simulink model "sim_tcyb_2023_obs"  (R2020a)
settings: Solver=ode4  StartTime=0.0  StopTime=30.0  FixedStep=0.01  RelTol=1e-3
values from neighbouring files (symbols this model uses):
  b1 = 6.0    (= 6)    [init_tcyb_2023_obs.m]
  c1 = 6.0    (= 6)    [init_tcyb_2023_obs.m]
  delta1 = 0.1    [init_tcyb_2023_obs.m]
  delta2 = 0.1    [init_tcyb_2023_obs.m]
  k0 = 2    [init_tcyb_2023_obs.m]
  kai_1_t = 0.02    [init_tcyb_2023_obs.m]
  kai_3_t = 0.1    [init_tcyb_2023_obs.m]
  lambda_max_P = max(eig(Pij))    [init_tcyb_2023_obs.m]
  lambda_min_Q = min(eig(Qij))    [init_tcyb_2023_obs.m]
  Mii = diag([1;0;0;0;1])    [init_tcyb_2023_obs.m]
  pos0 = zeros(3, 1)    [init_tcyb_2023_obs.m]
  PZ0 = P0(3)    [init_tcyb_2023_obs.m]
  PZ1 = 10    [init_tcyb_2023_obs.m]
  R0 = 4    [init_tcyb_2023_obs.m]
  R1 = 8    [init_tcyb_2023_obs.m]
  Rx2 = 10    [init_tcyb_2023_obs.m]
  Ry2 = 6    [init_tcyb_2023_obs.m]
  Rz2 = 4    [init_tcyb_2023_obs.m]
  T0 = 0    [init_tcyb_2023_obs.m]
  T1 = tseq1    (= 10)    [init_tcyb_2023_obs.m]
  T12 = tseq1 + tseq12    (= 20)    [init_tcyb_2023_obs.m]
  T2 = tseq1 + tseq12 + tseq2    (= 30)    [init_tcyb_2023_obs.m]
  theta0 = ( 2 / 5 ) * pi    (= 1.25663706144)    [init_tcyb_2023_obs.m]
  ts1 = 10    [init_tcyb_2023_obs.m]
  ts2 = 20    [init_tcyb_2023_obs.m]
  vel0 = zeros(3, 1)    [init_tcyb_2023_obs.m]
  Wij = [0,0,1,0,0;              0,0,1,1,0;              1,0,0,0,1;              0,1,1,0,0;              0,0,1,0,0]    [init_tcyb_2023_obs.m]
  X1 = 8    [init_tcyb_2023_obs.m]
  X2 = 2    [init_tcyb_2023_obs.m]
  X3 = 3    [init_tcyb_2023_obs.m]
  Y1 = 10    [init_tcyb_2023_obs.m]
  Y2 = 2    [init_tcyb_2023_obs.m]
  Y3 = 4    [init_tcyb_2023_obs.m]
  Z1 = 4    [init_tcyb_2023_obs.m]
  Z2 = -6    [init_tcyb_2023_obs.m]
  Z3 = 2    [init_tcyb_2023_obs.m]
(part 1 of 2)
settings Model: Creator=zzy  LastModifiedBy=Hershey.A
settings DataIOCC: ReturnWorkspaceOutputs=off
settings DebuggingCC: ArithmeticOperatorsInVariantConditions=warning
settings SFSimCC: SimUseLocalCustomCode=off  CustomCodeUndefinedFunction=UseInterfaceOnly
settings RTWCC: RTWUseLocalCustomCode=off

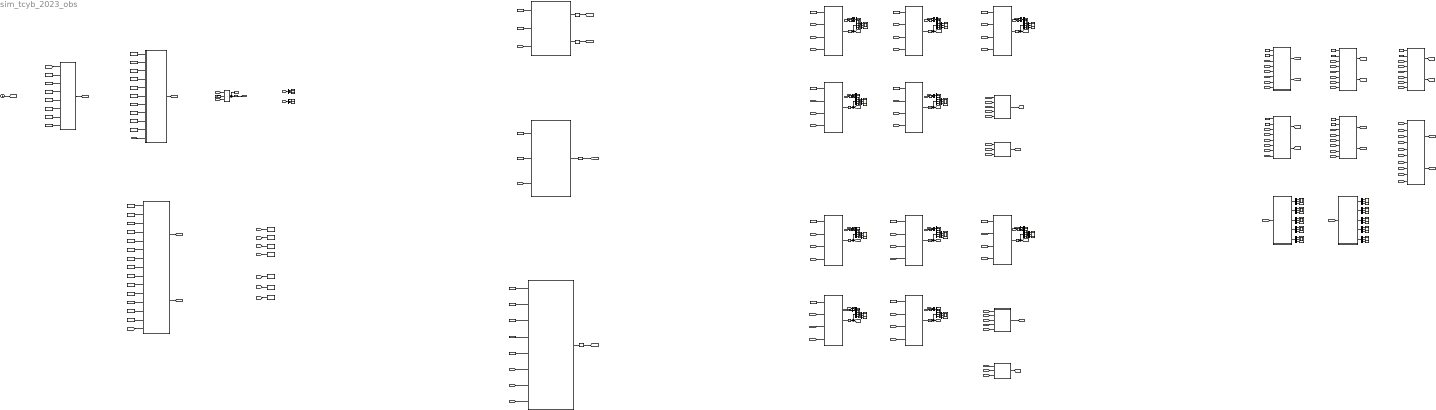
== system sim_tcyb_2023_obs ==
  Add{,1..9} (10 alike) : Sum
  Clock : Clock
  Constant : Constant  Value=T1
  Constant1 : Constant  Value=ts1
  Constant{10..14} (5 alike) : Constant  Value=c1
  Constant129 : Constant  Value=R0
  Constant130 : Constant  Value=R1
  Constant131 : Constant  Value=T0
  Constant132 : Constant  Value=Rz2
  Constant133 : Constant  Value=Ry2
  Constant134 : Constant  Value=Rx2
  Constant135 : Constant  Value=X1
  Constant136 : Constant  Value=X2
  Constant137 : Constant  Value=Y1
  Constant138 : Constant  Value=Y2
  Constant{15..19} (5 alike) : Constant  Value=b1
  Constant2 : Constant  Value=ts2
  Constant20 : Constant  Value=Z1
  Constant21 : Constant  Value=Z2
  Constant22 : Constant  Value=theta0
  Constant{223,227,232,236,240} (5 alike) : Constant  Value=Wij
  Constant{224,228,233,237,242} (5 alike) : Constant  Value=Mii
  Constant23 : Constant  Value=Z3
  Constant24 : Constant  Value=Y3
  Constant25 : Constant  Value=kai_1_t
  Constant26 : Constant  Value=X3
  Constant27 : Constant  Value=kai_3_t
  Constant28 : Constant  Value=T1
  Constant29 : Constant  Value=T12
  Constant3 : Constant  Value=k0
  Constant4 : Constant  Value=ts1
  Constant5 : Constant  Value=ts2
  Constant6 : Constant  Value=delta1
  Constant64 : Constant  Value=T2
  Constant65 : Constant  Value=R0
  Constant66 : Constant  Value=R1
  Constant67 : Constant  Value=Rx2
  Constant68 : Constant  Value=Ry2
  Constant69 : Constant  Value=Rz2
  Constant7 : Constant  Value=delta2
  Constant70 : Constant  Value=T2
  Constant71 : Constant  Value=T1
  Constant72 : Constant  Value=PZ0
  Constant73 : Constant  Value=PZ1
  Constant8 : Constant  Value=lambda_max_P
  Constant9 : Constant  Value=lambda_min_Q
  Demux{1,22,68..97} (32 alike) : Demux  Outputs=3
  Memory{,1..3} (4 alike) : Memory
  Mux{86..108,119,130..135} (30 alike) : Mux  Inputs=2
  Selector1 : Selector  NumberOfDimensions=2  InputPortWidth=3  IndexOptions=Index vector (dialog),Index vector (dialog)  Indices=[1 2 3],4  OutputSizes=1,1
  Selector10 : Selector  NumberOfDimensions=2  InputPortWidth=3  IndexOptions=Index vector (dialog),Index vector (dialog)  Indices=[1 2 3],5  OutputSizes=1,1
  Selector2 : Selector  NumberOfDimensions=2  InputPortWidth=3  IndexOptions=Index vector (dialog),Index vector (dialog)  Indices=[1 2 3],5  OutputSizes=1,1
  Selector3 : Selector  NumberOfDimensions=2  InputPortWidth=3  IndexOptions=Index vector (dialog),Index vector (dialog)  Indices=[1 2 3],3  OutputSizes=1,1
  Selector4 : Selector  NumberOfDimensions=2  InputPortWidth=3  IndexOptions=Index vector (dialog),Index vector (dialog)  Indices=[1 2 3],1  OutputSizes=1,1
  Selector5 : Selector  NumberOfDimensions=2  InputPortWidth=3  IndexOptions=Index vector (dialog),Index vector (dialog)  Indices=[1 2 3],2  OutputSizes=1,1
  Selector6 : Selector  NumberOfDimensions=2  InputPortWidth=3  IndexOptions=Index vector (dialog),Index vector (dialog)  Indices=[1 2 3],1  OutputSizes=1,1
  Selector7 : Selector  NumberOfDimensions=2  InputPortWidth=3  IndexOptions=Index vector (dialog),Index vector (dialog)  Indices=[1 2 3],2  OutputSizes=1,1
  Selector8 : Selector  NumberOfDimensions=2  InputPortWidth=3  IndexOptions=Index vector (dialog),Index vector (dialog)  Indices=[1 2 3],3  OutputSizes=1,1
  Selector9 : Selector  NumberOfDimensions=2  InputPortWidth=3  IndexOptions=Index vector (dialog),Index vector (dialog)  Indices=[1 2 3],4  OutputSizes=1,1
  Step : Step  Time=T1+0.01  SampleTime=0
  To Workspace : ToWorkspace  VariableName=eta_d_est_vec  SampleTime=-1
  To Workspace17 : ToWorkspace  VariableName=ksi_est_err  SampleTime=-1
  To Workspace18 : ToWorkspace  VariableName=ksi_d_est_vec  SampleTime=-1
  To Workspace22 : ToWorkspace  VariableName=eta_est_err  SampleTime=-1
  To Workspace3 : ToWorkspace  VariableName=u0  SampleTime=-1
  To Workspace4 : ToWorkspace  VariableName=eta0  SampleTime=-1
  To Workspace5 : ToWorkspace  VariableName=ksi0  SampleTime=-1
  cal lumped observation error agent 1 : MATLAB Function  TreatAsAtomicUnit=on
  cal lumped observation error agent 2 : MATLAB Function  TreatAsAtomicUnit=on
  cal lumped observation error agent 3 : MATLAB Function  TreatAsAtomicUnit=on
  cal lumped observation error agent 4 : MATLAB Function  TreatAsAtomicUnit=on
  cal lumped observation error agent 5 : MATLAB Function  TreatAsAtomicUnit=on
  cal position estimate error : MATLAB Function  TreatAsAtomicUnit=on
  cal velocity estimate error : MATLAB Function  TreatAsAtomicUnit=on
  combine follower desire velocity estimaters : MATLAB Function  TreatAsAtomicUnit=on
  combine leader position estimaters : MATLAB Function  TreatAsAtomicUnit=on
  "combine lumped follower observation error " : MATLAB Function  TreatAsAtomicUnit=on
  distributed follower desire position observer agent 1 : MATLAB Function  TreatAsAtomicUnit=on
  distributed follower desire position observer agent 2 : MATLAB Function  TreatAsAtomicUnit=on
  distributed follower desire position observer agent 3 : MATLAB Function  TreatAsAtomicUnit=on
  distributed follower desire position observer agent 4 : MATLAB Function  TreatAsAtomicUnit=on
  distributed follower desire position observer agent 5 : MATLAB Function  TreatAsAtomicUnit=on
  distributed follower desire velocity observer agent 1 : MATLAB Function  TreatAsAtomicUnit=on
  distributed follower desire velocity observer agent 2 : MATLAB Function  TreatAsAtomicUnit=on
  distributed follower desire velocity observer agent 3 : MATLAB Function  TreatAsAtomicUnit=on
  distributed follower desire velocity observer agent 4 : MATLAB Function  TreatAsAtomicUnit=on
  distributed follower desire velocity observer agent 5 : MATLAB Function  TreatAsAtomicUnit=on
  divide eta_est_err : MATLAB Function  TreatAsAtomicUnit=on
  divide ksi_est_err : MATLAB Function  TreatAsAtomicUnit=on
  eta_0 : Scope  NumInputPorts=3
  eta_d_est_{1..5} (5 alike) : Scope  NumInputPorts=3
  eta_est_err_{1..5} (5 alike) : Scope  NumInputPorts=3
  generate function eta_t : MATLAB Function  TreatAsAtomicUnit=on
  generate function h_t : MATLAB Function  TreatAsAtomicUnit=on
  generate function ksy_t d_ksy_t : MATLAB Function  TreatAsAtomicUnit=on
  ksi_0 : Scope  NumInputPorts=3
  ksi_d_est_{1..5} (5 alike) : Scope  NumInputPorts=3
  ksi_est_err_{1..5} (5 alike) : Scope  NumInputPorts=3
  leader control input : MATLAB Function  TreatAsAtomicUnit=on
  leader eta0 Integrator : Integrator  ExternalReset=rising  InitialConditionSource=external  InitialCondition=vel0
  leader ksi0 Integrator : Integrator  InitialCondition=pos0
  position observe Integrator {1..5} (5 alike) : Integrator  InitialCondition=zeros(3,1)
  process velocity : MATLAB Function  TreatAsAtomicUnit=on
  set desire formation configuration : MATLAB Function  TreatAsAtomicUnit=on
  velocity observe Integrator {1..5} (5 alike) : Integrator  InitialCondition=zeros(3,1)
  wires:
  [ksi0] -> cal lumped observation error agent 2/4(ksi0)
  Constant227/1 -> cal lumped observation error agent 2/1(wij)
  Add3/1 -> Demux76/1
  Add8/1 -> Demux97/1
  Mux134/1 -> ksi_d_est_3/2
  Mux135/1 -> ksi_d_est_3/3
  Demux93/2 -> Mux130/2
  position observe Integrator 2/1 -> [ksi_d_est_2], Demux92/1
  Demux95/3 -> Mux135/2
  [ksi0] -> cal lumped observation error agent 1/4(ksi0)
  Demux94/2 -> Mux134/1
  [ksi0] -> Add6/1
  velocity observe Integrator 5/1 -> [eta_d_est_5], Demux77/1
  Demux93/1 -> Mux119/2
  distributed follower desire position observer agent 2/1(d_ksi_d_est_2) -> position observe Integrator 2/1
  Demux93/3 -> Mux132/2
  Mux108/1 -> ksi_d_est_1/3
  Add6/1 -> Demux93/1
  Mux119/1 -> ksi_d_est_2/1
  Demux88/3 -> Mux108/2
  Demux88/1 -> Mux86/2
  Add5/1 -> Demux88/1
  [eta_est_err_tilt_3] -> "combine lumped follower observation error "/8(eta_est_err_tilt_3)
  Demux73/2 -> Mux100/1
  Add1/1 -> Demux72/1
  [ksi0] -> cal lumped observation error agent 3/4(ksi0)
  [eta_d_est_vec] -> cal lumped observation error agent 1/6(eta_d_est_vec)
  [ksi_est_err_tilt_4] -> "combine lumped follower observation error "/4(ksi_est_err_tilt_4)
  Mux103/1 -> eta_d_est_4/2
  velocity observe Integrator 4/1 -> [eta_d_est_4], Demux75/1
  Demux77/2 -> Mux106/1
  Demux77/1 -> Mux105/1
  Mux107/1 -> eta_d_est_5/3
  distributed follower desire velocity observer agent 5/1(d_eta_d_est_5) -> velocity observe Integrator 5/1
  Mux104/1 -> eta_d_est_4/3
  Demux74/3 -> Mux101/2
  distributed follower desire velocity observer agent 3/1(d_eta_d_est_3) -> velocity observe Integrator 3/1
  Demux74/2 -> Mux100/2
  Demux75/2 -> Mux103/1
  Demux76/3 -> Mux104/2
  Demux75/3 -> Mux104/1
  cal lumped observation error agent 4/2(eta_est_err_tilt_4) -> [eta_est_err_tilt_4]
  Mux95/1 -> eta_d_est_2/1
  velocity observe Integrator 3/1 -> [eta_d_est_3], Demux73/1
  velocity observe Integrator 2/1 -> [eta_d_est_2], Demux71/1
  Demux72/1 -> Mux95/2
  [eta0] -> Add2/1
  [eta_est_err_tilt_5] -> "combine lumped follower observation error "/10(eta_est_err_tilt_5)
  Add/1 -> Demux70/1
  cal lumped observation error agent 2/1(ksi_est_err_tilt_2) -> [ksi_est_err_tilt_2]
  distributed follower desire velocity observer agent 2/1(d_eta_d_est_2) -> velocity observe Integrator 2/1
  Mux98/1 -> eta_d_est_2/3
  [eta_d_est_5] -> combine follower desire velocity estimaters/5(eta_d_est_5)
  cal lumped observation error agent 3/1(ksi_est_err_tilt_3) -> [ksi_est_err_tilt_3]
  Demux72/2 -> Mux96/2
  [ksi_d_est_vec] -> cal lumped observation error agent 5/3(ksi_d_est_vec)
  [eta_d_est_2] -> combine follower desire velocity estimaters/2(eta_d_est_2)
  Constant228/1 -> cal lumped observation error agent 2/2(w0)
  [ksi_est_err_tilt_2] -> "combine lumped follower observation error "/2(ksi_est_err_tilt_2)
  [ksi_est_err_tilt_5] -> "combine lumped follower observation error "/5(ksi_est_err_tilt_5)
  Demux76/1 -> Mux102/2
  cal lumped observation error agent 5/1(ksi_est_err_tilt_5) -> [ksi_est_err_tilt_5]
  [eta_est_err_tilt_2] -> "combine lumped follower observation error "/7(eta_est_err_tilt_2)
  [ksi_d_est_vec] -> cal lumped observation error agent 3/3(ksi_d_est_vec)
  Constant242/1 -> cal lumped observation error agent 5/2(w0)
  [ksi_d_est_vec] -> cal lumped observation error agent 4/3(ksi_d_est_vec)
  Mux105/1 -> eta_d_est_5/1
  [eta_est_err_tilt_4] -> "combine lumped follower observation error "/9(eta_est_err_tilt_4)
  Add7/1 -> Demux95/1
  Constant236/1 -> cal lumped observation error agent 4/1(wij)
  [eta0] -> cal lumped observation error agent 1/7(eta0)
  [eta0] -> cal lumped observation error agent 2/7(eta0)
  cal lumped observation error agent 1/2(eta_est_err_tilt_1) -> [eta_est_err_tilt_1]
  Demux77/3 -> Mux107/1
  cal lumped observation error agent 1/1(ksi_est_err_tilt_1) -> [ksi_est_err_tilt_1]
  [eta_d_est_vec] -> cal lumped observation error agent 2/6(eta_d_est_vec)
  cal lumped observation error agent 4/1(ksi_est_err_tilt_4) -> [ksi_est_err_tilt_4]
  Mux93/1 -> eta_d_est_1/2
  Demux69/2 -> Mux93/1
  Mux100/1 -> eta_d_est_3/2
  Mux94/1 -> eta_d_est_1/3
  Demux73/1 -> Mux99/1
  [ksi_d_est_3] -> combine leader position estimaters/3(ksi_d_est_3)
  Demux70/2 -> Mux93/2
  [eta0] -> Add/1
  [ksi0] -> cal position estimate error/2(ksi0)
  Demux69/3 -> Mux94/1
  distributed follower desire position observer agent 3/1(d_ksi_d_est_3) -> position observe Integrator 3/1
  [eta_d_est_4] -> combine follower desire velocity estimaters/4(eta_d_est_4)
  [eta_d_est_1] -> combine follower desire velocity estimaters/1(eta_d_est_1)
  Constant233/1 -> cal lumped observation error agent 3/2(w0)
  Demux78/1 -> Mux86/1
  Demux86/3 -> eta_est_err_1/3
  Demux89/2 -> eta_est_err_3/2
  Demux87/1 -> eta_est_err_2/1
  divide eta_est_err/2(eta_est_err_2) -> Demux87/1
  Demux85/2 -> ksi_est_err_5/2
  Demux90/1 -> eta_est_err_4/1
  Demux90/2 -> eta_est_err_4/2
  Mux86/1 -> ksi_d_est_1/1
  Mux130/1 -> ksi_d_est_2/2
  Demux87/2 -> eta_est_err_2/2
  Mux131/1 -> ksi_d_est_5/3
  distributed follower desire position observer agent 1/1(d_ksi_d_est_1) -> position observe Integrator 1/1
  Demux84/1 -> ksi_est_err_4/1
  divide eta_est_err/4(eta_est_err_4) -> Demux90/1
  position observe Integrator 5/1 -> [ksi_d_est_5], Demux68/1
  Demux85/3 -> ksi_est_err_5/3
  Constant224/1 -> cal lumped observation error agent 1/2(w0)
  Demux85/1 -> ksi_est_err_5/1
  Mux97/1 -> ksi_d_est_1/2
  Demux84/2 -> ksi_est_err_4/2
  Demux94/3 -> Mux135/1
  divide ksi_est_err/4(ksi_est_err_4) -> Demux84/1
  Mux89/1 -> ksi_d_est_4/3
  Demux82/3 -> ksi_est_err_2/3
  Demux92/2 -> Mux130/1
  Constant240/1 -> cal lumped observation error agent 5/1(wij)
  [eta0] -> Add3/1
  Demux83/3 -> ksi_est_err_3/3
  Demux86/2 -> eta_est_err_1/2
  Demux88/2 -> Mux97/2
  Demux81/1 -> ksi_est_err_1/1
  Demux82/2 -> ksi_est_err_2/2
  [ksi_d_est_5] -> combine leader position estimaters/5(ksi_d_est_5)
  divide ksi_est_err/2(ksi_est_err_2) -> Demux82/1
  Demux91/1 -> eta_est_err_5/1
  position observe Integrator 3/1 -> [ksi_d_est_3], Demux94/1
  divide ksi_est_err/1(ksi_est_err_1) -> Demux81/1
  Demux82/1 -> ksi_est_err_2/1
  Demux68/3 -> Mux131/1
  distributed follower desire position observer agent 5/1(d_ksi_d_est_5) -> position observe Integrator 5/1
  Demux78/2 -> Mux97/1
  [eta0] -> cal lumped observation error agent 5/7(eta0)
  Demux78/3 -> Mux108/1
  [eta_d_est_3] -> combine follower desire velocity estimaters/3(eta_d_est_3)
  [eta0] -> cal velocity estimate error/2(eta0)
  Mux91/1 -> ksi_d_est_5/2
  Demux71/2 -> Mux96/1
  [eta_d_est_vec] -> cal lumped observation error agent 5/6(eta_d_est_vec)
  [ksi0] -> Add7/1
  [ksi0] -> Add9/1
  [ksi_est_err_tilt_1] -> "combine lumped follower observation error "/1(ksi_est_err_tilt_1)
  distributed follower desire velocity observer agent 4/1(d_eta_d_est_4) -> velocity observe Integrator 4/1
  Mux90/1 -> ksi_d_est_5/1
  Constant223/1 -> cal lumped observation error agent 1/1(wij)
  [eta0] -> cal lumped observation error agent 3/7(eta0)
  Demux80/1 -> Mux90/2
  Mux88/1 -> ksi_d_est_4/2
  Add4/1 -> Demux79/1
  Constant232/1 -> cal lumped observation error agent 3/1(wij)
  Mux87/1 -> ksi_d_est_4/1
  position observe Integrator 1/1 -> [ksi_d_est_1], Demux78/1
  Demux80/3 -> Mux131/2
  [ksi0] -> cal lumped observation error agent 5/4(ksi0)
  [ksi_d_est_vec] -> cal position estimate error/1(ksi_d_est_vec)
  Demux73/3 -> Mux101/1
  Demux69/1 -> Mux92/1
  Demux96/2 -> Mux88/1
  position observe Integrator 4/1 -> [ksi_d_est_4], Demux96/1
  Demux72/3 -> Mux98/2
  Demux74/1 -> Mux99/2
  Constant237/1 -> cal lumped observation error agent 4/2(w0)
  Mux132/1 -> ksi_d_est_2/3
  Demux70/3 -> Mux94/2
  Demux71/1 -> Mux95/1
  Mux133/1 -> ksi_d_est_3/1
  [ksi0] -> Add8/1
  cal lumped observation error agent 3/2(eta_est_err_tilt_3) -> [eta_est_err_tilt_3]
  distributed follower desire position observer agent 4/1(d_ksi_d_est_4) -> position observe Integrator 4/1
  [eta_d_est_vec] -> cal velocity estimate error/1(eta_d_est_vec)
  Add2/1 -> Demux74/1
  Demux95/2 -> Mux134/2
  Demux97/1 -> Mux87/2
  [eta0] -> Add1/1
  [eta0] -> Add4/1
  [ksi0] -> cal lumped observation error agent 4/4(ksi0)
  distributed follower desire velocity observer agent 1/1(d_eta_d_est_1) -> velocity observe Integrator 1/1
  Demux96/1 -> Mux87/1
  [ksi_d_est_2] -> combine leader position estimaters/2(ksi_d_est_2)
  [ksi_d_est_vec] -> cal lumped observation error agent 1/3(ksi_d_est_vec)
  Demux97/2 -> Mux88/2
  Demux83/2 -> ksi_est_err_3/2
  [ksi_est_err_tilt_3] -> "combine lumped follower observation error "/3(ksi_est_err_tilt_3)
  Demux71/3 -> Mux98/1
  Demux86/1 -> eta_est_err_1/1
  Mux101/1 -> eta_d_est_3/3
  cal lumped observation error agent 2/2(eta_est_err_tilt_2) -> [eta_est_err_tilt_2]
  Demux87/3 -> eta_est_err_2/3
  Mux96/1 -> eta_d_est_2/2
  Demux79/3 -> Mux107/2
  cal lumped observation error agent 5/2(eta_est_err_tilt_5) -> [eta_est_err_tilt_5]
  [eta_est_err] -> divide eta_est_err/1(eta_est_err)
  velocity observe Integrator 1/1 -> [eta_d_est_1], Demux69/1
  [ksi_d_est_4] -> combine leader position estimaters/4(ksi_d_est_4)
  Demux76/2 -> Mux103/2
  Demux79/2 -> Mux106/2
  [eta0] -> cal lumped observation error agent 4/7(eta0)
  divide ksi_est_err/3(ksi_est_err_3) -> Demux83/1
  Demux95/1 -> Mux133/2
  divide eta_est_err/5(eta_est_err_5) -> Demux91/1
  Demux96/3 -> Mux89/1
  Demux92/1 -> Mux119/1
  Mux99/1 -> eta_d_est_3/1
  Demux89/1 -> eta_est_err_3/1
  Demux83/1 -> ksi_est_err_3/1
  Demux81/3 -> ksi_est_err_1/3
  Add9/1 -> Demux80/1
  Mux102/1 -> eta_d_est_4/1
  Demux68/1 -> Mux90/1
  Demux80/2 -> Mux91/2
  Demux92/3 -> Mux132/1
  [eta_est_err_tilt_1] -> "combine lumped follower observation error "/6(eta_est_err_tilt_1)
  [ksi_est_err] -> divide ksi_est_err/1(ksi_est_err)
  Demux68/2 -> Mux91/1
  Demux91/3 -> eta_est_err_5/3
  [ksi0] -> Add5/1
  [ksi_d_est_1] -> combine leader position estimaters/1(ksi_d_est_1)
  [ksi_d_est_vec] -> cal lumped observation error agent 2/3(ksi_d_est_vec)
  Demux94/1 -> Mux133/1
  divide eta_est_err/3(eta_est_err_3) -> Demux89/1
  Demux89/3 -> eta_est_err_3/3
  divide ksi_est_err/5(ksi_est_err_5) -> Demux85/1
  Demux79/1 -> Mux105/2
  [eta_d_est_vec] -> cal lumped observation error agent 3/6(eta_d_est_vec)
  Demux81/2 -> ksi_est_err_1/2
  Demux84/3 -> ksi_est_err_4/3
  Demux70/1 -> Mux92/2
  Demux91/2 -> eta_est_err_5/2
  Demux90/3 -> eta_est_err_4/3
  [eta_d_est_vec] -> cal lumped observation error agent 4/6(eta_d_est_vec)
  Demux75/1 -> Mux102/1
  divide eta_est_err/1(eta_est_err_1) -> Demux86/1
  Mux106/1 -> eta_d_est_5/2
  Demux97/3 -> Mux89/2
  Mux92/1 -> eta_d_est_1/1
  cal position estimate error/1(ksi_est_err) -> [ksi_est_err]
  cal velocity estimate error/1(eta_est_err) -> [eta_est_err]
  combine leader position estimaters/1(ksi_d_est_vec) -> [ksi_d_est_vec]
  combine follower desire velocity estimaters/1(eta_d_est_vec) -> [eta_d_est_vec]
  "combine lumped follower observation error "/1(ksi_est_err_tilt_vec) -> [ksi_est_err_tilt_vec]
  "combine lumped follower observation error "/2(eta_est_err_tilt_vec) -> [eta_est_err_tilt_vec]
  [tsim] -> generate function ksy_t d_ksy_t/3(tsim)
  Constant1/1 -> generate function ksy_t d_ksy_t/1(ts1)
  Constant2/1 -> generate function ksy_t d_ksy_t/2(ts2)
  generate function ksy_t d_ksy_t/1(ksy_t) -> Memory/1
  Memory/1 -> [ksy_t]
  Memory1/1 -> [d_ksy_t]
  generate function ksy_t d_ksy_t/2(d_ksy_t) -> Memory1/1
  Constant3/1 -> generate function h_t/1(k0)
  Constant4/1 -> generate function h_t/2(ts1)
  Constant5/1 -> generate function h_t/3(ts2)
  [tsim] -> generate function h_t/6(tsim)
  Constant6/1 -> generate function h_t/4(delta1)
  Constant7/1 -> generate function h_t/5(delta2)
  [ksy_t] -> generate function h_t/7(ksy_t)
  [d_ksy_t] -> generate function h_t/8(d_ksy_t)
  Memory2/1 -> [h_t]
  generate function h_t/1(h_t) -> Memory2/1
  Constant8/1 -> generate function eta_t/1(lambda_max_P)
  Constant9/1 -> generate function eta_t/2(lambda_min_Q)
  [h_t] -> generate function eta_t/3(h_t)
  Memory3/1 -> [eta_t]
  generate function eta_t/1(eta_t) -> Memory3/1
  Constant10/1 -> distributed follower desire velocity observer agent 1/1(c1)
  [eta_t] -> distributed follower desire velocity observer agent 1/2(eta_t)
  [eta_est_err_tilt_vec] -> distributed follower desire velocity observer agent 1/4(eta_est_err_tilt_vec)
  Constant11/1 -> distributed follower desire velocity observer agent 2/1(c1)
  [eta_t] -> distributed follower desire velocity observer agent 2/2(eta_t)
  [eta_est_err_tilt_vec] -> distributed follower desire velocity observer agent 2/4(eta_est_err_tilt_vec)
  [eta_est_err_tilt_vec] -> distributed follower desire velocity observer agent 3/4(eta_est_err_tilt_vec)
  [eta_t] -> distributed follower desire velocity observer agent 3/2(eta_t)
  Constant12/1 -> distributed follower desire velocity observer agent 3/1(c1)
  Constant13/1 -> distributed follower desire velocity observer agent 4/1(c1)
  [eta_t] -> distributed follower desire velocity observer agent 4/2(eta_t)
  [eta_est_err_tilt_vec] -> distributed follower desire velocity observer agent 4/4(eta_est_err_tilt_vec)
  Constant14/1 -> distributed follower desire velocity observer agent 5/1(c1)
  [eta_t] -> distributed follower desire velocity observer agent 5/2(eta_t)
  [eta_est_err_tilt_vec] -> distributed follower desire velocity observer agent 5/4(eta_est_err_tilt_vec)
  Constant15/1 -> distributed follower desire position observer agent 1/1(b1)
  [ksi_est_err_tilt_vec] -> distributed follower desire position observer agent 1/3(ksi_est_err_tilt_vec)
  [eta_t] -> distributed follower desire position observer agent 1/2(eta_t)
  [eta_d_est_vec] -> distributed follower desire position observer agent 1/4(eta_d_est_vec)
  Constant16/1 -> distributed follower desire position observer agent 2/1(b1)
  [eta_t] -> distributed follower desire position observer agent 2/2(eta_t)
  [ksi_est_err_tilt_vec] -> distributed follower desire position observer agent 2/3(ksi_est_err_tilt_vec)
  [eta_d_est_vec] -> distributed follower desire position observer agent 2/4(eta_d_est_vec)
  Constant17/1 -> distributed follower desire position observer agent 3/1(b1)
  [eta_t] -> distributed follower desire position observer agent 3/2(eta_t)
  [ksi_est_err_tilt_vec] -> distributed follower desire position observer agent 3/3(ksi_est_err_tilt_vec)
  [eta_d_est_vec] -> distributed follower desire position observer agent 3/4(eta_d_est_vec)
  Constant18/1 -> distributed follower desire position observer agent 4/1(b1)
  [eta_t] -> distributed follower desire position observer agent 4/2(eta_t)
  [ksi_est_err_tilt_vec] -> distributed follower desire position observer agent 4/3(ksi_est_err_tilt_vec)
  [eta_d_est_vec] -> distributed follower desire position observer agent 4/4(eta_d_est_vec)
  Constant19/1 -> distributed follower desire position observer agent 5/1(b1)
  [eta_t] -> distributed follower desire position observer agent 5/2(eta_t)
  [ksi_est_err_tilt_vec] -> distributed follower desire position observer agent 5/3(ksi_est_err_tilt_vec)
  [eta_d_est_vec] -> distributed follower desire position observer agent 5/4(eta_d_est_vec)
  Selector2/1 -> Add4/2
  [delta_eta_vec] -> Selector2/1
  [delta_eta_vec] -> Selector1/1
  Selector1/1 -> Add3/2
  [delta_eta_vec] -> Selector3/1
  Selector3/1 -> Add2/2
  [delta_eta_vec] -> Selector4/1
  Selector4/1 -> Add/2
  [delta_eta_vec] -> Selector5/1
  Selector5/1 -> Add1/2
  Constant28/1 -> set desire formation configuration/13(T1)
  Constant72/1 -> process velocity/4(PZ0)
  leader ksi0 Integrator/1 -> [ksi0]
  Constant70/1 -> process velocity/3(T2)
  [tsim] -> set desire formation configuration/15(t)
  Constant20/1 -> set desire formation configuration/7(Z1)
  [tsim] -> leader control input/1(t)
  Step/1 -> leader eta0 Integrator/2
  Demux1/2 -> ksi_0/2
  Constant129/1 -> process velocity/6(R0)
  Constant/1 -> leader control input/2(T1)
  Constant22/1 -> set desire formation configuration/10(theta0)
  set desire formation configuration/2(delta_eta_vec) -> [delta_eta_vec]
  Constant71/1 -> process velocity/2(T1)
  Constant138/1 -> set desire formation configuration/5(Y2)
  Constant21/1 -> set desire formation configuration/8(Z2)
  set desire formation configuration/1(delta_ksi_vec) -> [delta_ksi_vec]
  Constant24/1 -> set desire formation configuration/6(Y3)
  Constant132/1 -> process velocity/10(Rz2)
  Demux22/1 -> eta_0/1
  [V_init_out] -> leader eta0 Integrator/3
  Constant68/1 -> leader control input/7(Ry2)
  Demux1/3 -> ksi_0/3
  Constant25/1 -> set desire formation configuration/11(kai_1_t)
  Demux22/2 -> eta_0/2
  Constant29/1 -> set desire formation configuration/14(T12)
  [tsim] -> process velocity/11(t)
  Constant135/1 -> set desire formation configuration/1(X1)
  Constant23/1 -> set desire formation configuration/9(Z3)
  [eta0] -> Demux22/1
  Constant133/1 -> process velocity/9(Ry2)
  Constant73/1 -> process velocity/5(PZ1)
  Demux1/1 -> ksi_0/1
  process velocity/1(V_init_out) -> [V_init_out]
  Demux22/3 -> eta_0/3
  Constant65/1 -> leader control input/4(R0)
  leader eta0 Integrator/1 -> [eta0], leader ksi0 Integrator/1
  Constant67/1 -> leader control input/6(Rx2)
  [ksi0] -> Demux1/1
  Clock/1 -> [tsim]
  Constant131/1 -> process velocity/1(T0)
  Constant137/1 -> set desire formation configuration/4(Y1)
  leader control input/1(u0) -> [u0]
  Constant64/1 -> leader control input/3(T2)
  Constant130/1 -> process velocity/7(R1)
  [u0] -> leader eta0 Integrator/1
  Constant134/1 -> process velocity/8(Rx2)
  Constant26/1 -> set desire formation configuration/3(X3)
  Constant66/1 -> leader control input/5(R1)
  Constant27/1 -> set desire formation configuration/12(kai_3_t)
  Constant69/1 -> leader control input/8(Rz2)
  Constant136/1 -> set desire formation configuration/2(X2)
  [ksi_est_err] -> To Workspace17/1
  [u0] -> To Workspace3/1
  [eta_est_err] -> To Workspace22/1
  [ksi_d_est_vec] -> To Workspace18/1
  [ksi0] -> To Workspace5/1
  [eta_d_est_vec] -> To Workspace/1
  [eta0] -> To Workspace4/1
  [delta_ksi_vec] -> cal lumped observation error agent 2/5(delta_ksi_vec)
  [delta_ksi_vec] -> Selector6/1
  Selector6/1 -> Add5/2
  [delta_ksi_vec] -> Selector7/1
  Selector7/1 -> Add6/2
  [delta_ksi_vec] -> Selector8/1
  Selector8/1 -> Add7/2
  [delta_ksi_vec] -> Selector9/1
  Selector9/1 -> Add8/2
  [delta_ksi_vec] -> Selector10/1
  Selector10/1 -> Add9/2
  [delta_ksi_vec] -> cal lumped observation error agent 1/5(delta_ksi_vec)
  [delta_eta_vec] -> cal lumped observation error agent 1/8(delta_eta_vec)
  [delta_ksi_vec] -> cal lumped observation error agent 3/5(delta_ksi_vec)
  [delta_eta_vec] -> cal lumped observation error agent 3/8(delta_eta_vec)
  [delta_ksi_vec] -> cal lumped observation error agent 5/5(delta_ksi_vec)
  [delta_eta_vec] -> cal lumped observation error agent 5/8(delta_eta_vec)
  [delta_eta_vec] -> cal lumped observation error agent 2/8(delta_eta_vec)
  [delta_ksi_vec] -> cal lumped observation error agent 4/5(delta_ksi_vec)
  [delta_eta_vec] -> cal lumped observation error agent 4/8(delta_eta_vec)
  [u0] -> distributed follower desire velocity observer agent 1/3(u0)
  [u0] -> distributed follower desire velocity observer agent 2/3(u0)
  [u0] -> distributed follower desire velocity observer agent 3/3(u0)
  [u0] -> distributed follower desire velocity observer agent 4/3(u0)
  [u0] -> distributed follower desire velocity observer agent 5/3(u0)
  [delta_ksi_vec] -> cal position estimate error/3(delta_ksi_vec)
  [delta_eta_vec] -> cal velocity estimate error/3(delta_eta_vec)

== matlab function sim_tcyb_2023_obs/set desire formation configuration ==
  data: X1 input; X2 input; X3 input; Y1 input; Y2 input; Y3 input; Z1 input; Z2 input; Z3 input; theta0 input; kai_1_t input; kai_3_t input; T1 input; T12 input; t input; delta_ksi_vec output; delta_eta_vec output
function [delta_ksi_vec, delta_eta_vec] = fcn(X1, X2, X3, Y1, Y2, Y3, Z1, Z2, Z3, theta0, ...
                                                                                    kai_1_t, kai_3_t, T1, T12, t)
%%%% 计算跟随者期望速度分布式观测器误差
delta_ksi_vec = zeros(3, 5);
delta_eta_vec = zeros(3, 5);
if t <= ( T1 + 1e-04 )
    exp_tmp = exp( -kai_1_t * t );
    delta_ksi_vec(:, 1) = [ X1 * cos( theta0 ) - X2 * exp_tmp; ...
                                            Y1 * sin( theta0 ) - Y2 * exp_tmp; ...
                                            Z1 - Z2 * exp_tmp ];
    delta_ksi_vec(:, 2) = [ - X1 * cos( theta0 ) + X2 * exp_tmp; ...
                                            Y1 * sin( theta0 ) - Y2 * exp_tmp; ...
                                            Z1 + Z2 * exp_tmp ];
    delta_ksi_vec(:, 3) = [ X1 - X2 * exp_tmp; ...
                                            Y2 * exp_tmp; ...
                                            ( 3 / 8 ) * Z1 + Z2 * exp_tmp ];
    delta_ksi_vec(:, 4) = [ - X1 * cos( theta0 ) + X2 * exp_tmp; ...
                                            - Y1 * sin( theta0 ) + Y2 * exp_tmp; ...
                                            Z1 + Z2 * exp_tmp ];
    delta_ksi_vec(:, 5) = [ X1 * cos( theta0 ) - X2 * exp_tmp; ...
                                            - Y1 * sin( theta0 ) + Y2 * exp_tmp; ...
                                            Z1 - Z2 * exp_tmp ];
    delta_eta_vec(:, 1) = [ kai_1_t * X2 * exp_tmp; kai_1_t * Y2 * exp_tmp; kai_1_t * Z2 * exp_tmp ];
    delta_eta_vec(:, 2) = [ - kai_1_t * X2 * exp_tmp; kai_1_t * Y2 * exp_tmp; - kai_1_t * Z2 * exp_tmp ];
    delta_eta_vec(:, 3) = [ kai_1_t * X2 * exp_tmp; - kai_1_t * Y2 * exp_tmp; - kai_1_t * Z2 * exp_tmp ];
    delta_eta_vec(:, 4) = [ - kai_1_t * X2 * exp_tmp; - kai_1_t * Y2 * exp_tmp; - kai_1_t * Z2 * exp_tmp ];
    delta_eta_vec(:, 5) = [ kai_1_t * X2 * exp_tmp; - kai_1_t * Y2 * exp_tmp; kai_1_t * Z2 * exp_tmp ];
elseif t <= ( T12 + 1e-04 )
    delta_ksi_vec(:, 1) = [ X1 * cos( theta0 ) - X2; Y1 * sin( theta0 ) - Y2; Z1 - Z2 ];
    delta_ksi_vec(:, 2) = [ - X1 * cos( theta0 ) + X2; Y1 * sin( theta0 ) - Y2; Z1 + Z2 ];
    delta_ksi_vec(:, 3) = [ X1 - X2; 0; ( 3 / 8 ) * Z1 + Z2 ];
    delta_ksi_vec(:, 4) = [ - X1 * cos( theta0 ) + X2; - Y1 * sin( theta0 ) + Y2; Z1 + Z2 ];
    delta_ksi_vec(:, 5) = [ X1 * cos( theta0 ) - X2; - Y1 * sin( theta0 ) + Y2; Z1 - Z2 ];
else
    exp_tmp = 1 / ( 1 + exp( - kai_3_t * ( t - T12 - 5 ) ) );
    tmp_2 = exp( - kai_3_t * ( t - T12 - 5 ) ) / ( ( 1 + exp( - kai_3_t * ( t - T12 - 5 ) ) ) ^ 2 );
    delta_ksi_vec(:, 1) = [ X1 * cos( theta0 ) - X2 + X3 * exp_tmp; ...
                                            Y1 * sin( theta0 ) - Y2 + Y3 * exp_tmp; ...
                                            Z1 - Z2 + Z3 * exp_tmp ];
    delta_ksi_vec(:, 2) = [ - X1 * cos( theta0 ) + X2 - X3 * exp_tmp; ...
                                            Y1 * sin( theta0 ) - Y2 + Y3 * exp_tmp; ...
                                            Z1 + Z2 - Z3 * exp_tmp ];
    delta_ksi_vec(:, 3) = [ X1 - X2 + X3 * exp_tmp; ...
                                            - Y3 * exp_tmp; ...
                                            ( 3 / 8 ) * Z1 + Z2 - Z3 * exp_tmp ];
    delta_ksi_vec(:, 4) = [ - X1 * cos( theta0 ) + X2 - X3 * exp_tmp; ...
                                            - Y1 * sin( theta0 ) + Y2 - Y3 * exp_tmp; ...
                                            Z1 + Z2 - Z3 * exp_tmp ];
    delta_ksi_vec(:, 5) = [ X1 * cos( theta0 ) - X2 + X3 * exp_tmp; ...
                                            - Y1 * sin( theta0 ) + Y2 - Y3 * exp_tmp; ...
                                            Z1 - Z2 + Z3 * exp_tmp ];
    delta_eta_vec(:, 1) = [ kai_3_t * X3 * tmp_2; kai_3_t * Y3 * tmp_2; kai_3_t * Z3 * tmp_2 ];
    delta_eta_vec(:, 2) = [ - kai_3_t * X3 * tmp_2; kai_3_t * Y3 * tmp_2; kai_3_t * Z3 * tmp_2 ];
    delta_eta_vec(:, 3) = [ kai_3_t * X3 * tmp_2; - kai_3_t * Y3 * tmp_2; - kai_3_t * Z3 * tmp_2 ];
    delta_eta_vec(:, 4) = [ - kai_3_t * X3 * tmp_2; - kai_3_t * Y3 * tmp_2; - kai_3_t * Z3 * tmp_2 ];
    delta_eta_vec(:, 5) = [ kai_3_t * X3 * tmp_2; kai_3_t * Y3 * tmp_2; - kai_3_t * Z3 * tmp_2 ];
end

== matlab function sim_tcyb_2023_obs/distributed follower desire velocity observer agent 2 ==
  data: c1 input; d_eta_d_est_2 output; eta_t input; u0 input; eta_est_err_tilt_vec input
function d_eta_d_est_2 = fcn(c1, eta_t, u0, eta_est_err_tilt_vec)
%%%% 跟随者期望速度分布式观测器
iiuav = 2;
d_eta_d_est_2 = u0(:) - 2 * ( eta_t + 2 ) * eta_est_err_tilt_vec(:,iiuav) ...
                                - c1 * ( eta_t + 2 ) * sign( eta_est_err_tilt_vec(:,iiuav) );

== matlab function sim_tcyb_2023_obs/distributed follower desire velocity observer agent 3 ==
  data: c1 input; d_eta_d_est_3 output; eta_t input; u0 input; eta_est_err_tilt_vec input
function d_eta_d_est_3 = fcn(c1, eta_t, u0, eta_est_err_tilt_vec)
%%%% 跟随者期望速度分布式观测器
iiuav = 3;
d_eta_d_est_3 = u0(:) - 2 * ( eta_t + 2 ) * eta_est_err_tilt_vec(:,iiuav) ...
                                - c1 * ( eta_t + 2 ) * sign( eta_est_err_tilt_vec(:,iiuav) );

== matlab function sim_tcyb_2023_obs/distributed follower desire velocity observer agent 4 ==
  data: c1 input; d_eta_d_est_4 output; eta_t input; u0 input; eta_est_err_tilt_vec input
function d_eta_d_est_4 = fcn(c1, eta_t, u0, eta_est_err_tilt_vec)
%%%% 跟随者期望速度分布式观测器
iiuav = 4;
d_eta_d_est_4 = u0(:) - 2 * ( eta_t + 2 ) * eta_est_err_tilt_vec(:,iiuav) ...
                                - c1 * ( eta_t + 2 ) * sign( eta_est_err_tilt_vec(:,iiuav) );

== matlab function sim_tcyb_2023_obs/distributed follower desire velocity observer agent 5 ==
  data: c1 input; d_eta_d_est_5 output; eta_t input; u0 input; eta_est_err_tilt_vec input
function d_eta_d_est_5 = fcn(c1, eta_t, u0, eta_est_err_tilt_vec)
%%%% 跟随者期望速度分布式观测器
iiuav = 5;
d_eta_d_est_5 = u0(:) - 2 * ( eta_t + 2 ) * eta_est_err_tilt_vec(:,iiuav) ...
                                - c1 * ( eta_t + 2 ) * sign( eta_est_err_tilt_vec(:,iiuav) );

== matlab function sim_tcyb_2023_obs/distributed follower desire position observer agent 1 ==
  data: b1 input; d_ksi_d_est_1 output; eta_t input; ksi_est_err_tilt_vec input; eta_d_est_vec input
function d_ksi_d_est_1 = fcn(b1, eta_t, ksi_est_err_tilt_vec, eta_d_est_vec)
%%%% 跟随者期望速度分布式观测器
iiuav = 1;
d_ksi_d_est_1 = eta_d_est_vec(:,iiuav) - 2 * ( eta_t + 2 ) * ksi_est_err_tilt_vec(:,iiuav) ...
                                - b1 * ( eta_t + 2 ) * sign( ksi_est_err_tilt_vec(:,iiuav) );

== matlab function sim_tcyb_2023_obs/distributed follower desire position observer agent 2 ==
  data: b1 input; d_ksi_d_est_2 output; eta_t input; ksi_est_err_tilt_vec input; eta_d_est_vec input
function d_ksi_d_est_2 = fcn(b1, eta_t, ksi_est_err_tilt_vec, eta_d_est_vec)
%%%% 跟随者期望速度分布式观测器
iiuav = 2;
d_ksi_d_est_2 = eta_d_est_vec(:,iiuav) - 2 * ( eta_t + 2 ) * ksi_est_err_tilt_vec(:,iiuav) ...
                                - b1 * ( eta_t + 2 ) * sign( ksi_est_err_tilt_vec(:,iiuav) );

== matlab function sim_tcyb_2023_obs/distributed follower desire position observer agent 3 ==
  data: b1 input; d_ksi_d_est_3 output; eta_t input; ksi_est_err_tilt_vec input; eta_d_est_vec input
function d_ksi_d_est_3 = fcn(b1, eta_t, ksi_est_err_tilt_vec, eta_d_est_vec)
%%%% 跟随者期望速度分布式观测器
iiuav = 3;
d_ksi_d_est_3 = eta_d_est_vec(:,iiuav) - 2 * ( eta_t + 2 ) * ksi_est_err_tilt_vec(:,iiuav) ...
                                - b1 * ( eta_t + 2 ) * sign( ksi_est_err_tilt_vec(:,iiuav) );

== matlab function sim_tcyb_2023_obs/distributed follower desire position observer agent 4 ==
  data: b1 input; d_ksi_d_est_4 output; eta_t input; ksi_est_err_tilt_vec input; eta_d_est_vec input
function d_ksi_d_est_4 = fcn(b1, eta_t, ksi_est_err_tilt_vec, eta_d_est_vec)
%%%% 跟随者期望速度分布式观测器
iiuav = 4;
d_ksi_d_est_4 = eta_d_est_vec(:,iiuav) - 2 * ( eta_t + 2 ) * ksi_est_err_tilt_vec(:,iiuav) ...
                                - b1 * ( eta_t + 2 ) * sign( ksi_est_err_tilt_vec(:,iiuav) );

== matlab function sim_tcyb_2023_obs/distributed follower desire position observer agent 5 ==
  data: b1 input; d_ksi_d_est_5 output; eta_t input; ksi_est_err_tilt_vec input; eta_d_est_vec input
function d_ksi_d_est_5 = fcn(b1, eta_t, ksi_est_err_tilt_vec, eta_d_est_vec)
%%%% 跟随者期望速度分布式观测器
iiuav = 5;
d_ksi_d_est_5 = eta_d_est_vec(:,iiuav) - 2 * ( eta_t + 2 ) * ksi_est_err_tilt_vec(:,iiuav) ...
                                - b1 * ( eta_t + 2 ) * sign( ksi_est_err_tilt_vec(:,iiuav) );

== matlab function sim_tcyb_2023_obs/cal lumped observation error agent 1 ==
  data: wij input; w0 input; ksi_d_est_vec input; ksi0 input; delta_ksi_vec input; eta_d_est_vec input; ksi_est_err_tilt_1 output; eta0 input; delta_eta_vec input; eta_est_err_tilt_1 output
function [ksi_est_err_tilt_1, eta_est_err_tilt_1]  = fcn(wij, w0, ksi_d_est_vec, ksi0, delta_ksi_vec, eta_d_est_vec, eta0, delta_eta_vec)
%%%% 计算跟随者期望速度分布式观测器误差
iiuav = 1;
ksi_est_err_tilt_1 = w0(iiuav, iiuav) * (ksi_d_est_vec(:,iiuav) - ksi0(:) - delta_ksi_vec(:,iiuav));
eta_est_err_tilt_1 = w0(iiuav, iiuav) * (eta_d_est_vec(:,iiuav) - eta0(:) - delta_eta_vec(:,iiuav));
for jjuav = 1:5
    ksi_est_err_tilt_1 = ksi_est_err_tilt_1 + ...
                                        wij(iiuav, jjuav) * ((ksi_d_est_vec(:,iiuav) - delta_ksi_vec(:,iiuav)) - (ksi_d_est_vec(:,jjuav) - delta_ksi_vec(:,jjuav)));
    eta_est_err_tilt_1 = eta_est_err_tilt_1 + ...
                                        wij(iiuav, jjuav) * ((eta_d_est_vec(:,iiuav) - delta_eta_vec(:,iiuav)) - (eta_d_est_vec(:,jjuav) - delta_eta_vec(:,jjuav)));
end

== matlab function sim_tcyb_2023_obs/cal lumped observation error agent 2 ==
  data: wij input; w0 input; ksi_d_est_vec input; ksi0 input; delta_ksi_vec input; eta_d_est_vec input; ksi_est_err_tilt_2 output; eta0 input; delta_eta_vec input; eta_est_err_tilt_2 output
function [ksi_est_err_tilt_2, eta_est_err_tilt_2]  = fcn(wij, w0, ksi_d_est_vec, ksi0, delta_ksi_vec, eta_d_est_vec, eta0, delta_eta_vec)
%%%% 计算跟随者期望速度分布式观测器误差
iiuav = 2;
ksi_est_err_tilt_2 = w0(iiuav, iiuav) * (ksi_d_est_vec(:,iiuav) - ksi0(:) - delta_ksi_vec(:,iiuav));
eta_est_err_tilt_2 = w0(iiuav, iiuav) * (eta_d_est_vec(:,iiuav) - eta0(:) - delta_eta_vec(:,iiuav));
for jjuav = 1:5
    ksi_est_err_tilt_2 = ksi_est_err_tilt_2 + ...
                                        wij(iiuav, jjuav) * ((ksi_d_est_vec(:,iiuav) - delta_ksi_vec(:,iiuav)) - (ksi_d_est_vec(:,jjuav) - delta_ksi_vec(:,jjuav)));
    eta_est_err_tilt_2 = eta_est_err_tilt_2 + ...
                                        wij(iiuav, jjuav) * ((eta_d_est_vec(:,iiuav) - delta_eta_vec(:,iiuav)) - (eta_d_est_vec(:,jjuav) - delta_eta_vec(:,jjuav)));
end

== matlab function sim_tcyb_2023_obs/cal lumped observation error agent 3 ==
  data: wij input; w0 input; ksi_d_est_vec input; ksi0 input; delta_ksi_vec input; eta_d_est_vec input; ksi_est_err_tilt_3 output; eta0 input; delta_eta_vec input; eta_est_err_tilt_3 output
function [ksi_est_err_tilt_3, eta_est_err_tilt_3]  = fcn(wij, w0, ksi_d_est_vec, ksi0, delta_ksi_vec, eta_d_est_vec, eta0, delta_eta_vec)
%%%% 计算跟随者期望速度分布式观测器误差
iiuav = 3;
ksi_est_err_tilt_3 = w0(iiuav, iiuav) * (ksi_d_est_vec(:,iiuav) - ksi0(:) - delta_ksi_vec(:,iiuav));
eta_est_err_tilt_3 = w0(iiuav, iiuav) * (eta_d_est_vec(:,iiuav) - eta0(:) - delta_eta_vec(:,iiuav));
for jjuav = 1:5
    ksi_est_err_tilt_3 = ksi_est_err_tilt_3 + ...
                                        wij(iiuav, jjuav) * ((ksi_d_est_vec(:,iiuav) - delta_ksi_vec(:,iiuav)) - (ksi_d_est_vec(:,jjuav) - delta_ksi_vec(:,jjuav)));
    eta_est_err_tilt_3 = eta_est_err_tilt_3 + ...
                                        wij(iiuav, jjuav) * ((eta_d_est_vec(:,iiuav) - delta_eta_vec(:,iiuav)) - (eta_d_est_vec(:,jjuav) - delta_eta_vec(:,jjuav)));
end

== matlab function sim_tcyb_2023_obs/cal lumped observation error agent 4 ==
  data: wij input; w0 input; ksi_d_est_vec input; ksi0 input; delta_ksi_vec input; eta_d_est_vec input; ksi_est_err_tilt_4 output; eta0 input; delta_eta_vec input; eta_est_err_tilt_4 output
function [ksi_est_err_tilt_4, eta_est_err_tilt_4]  = fcn(wij, w0, ksi_d_est_vec, ksi0, delta_ksi_vec, eta_d_est_vec, eta0, delta_eta_vec)
%%%% 计算跟随者期望速度分布式观测器误差
iiuav = 4;
ksi_est_err_tilt_4 = w0(iiuav, iiuav) * (ksi_d_est_vec(:,iiuav) - ksi0(:) - delta_ksi_vec(:,iiuav));
eta_est_err_tilt_4 = w0(iiuav, iiuav) * (eta_d_est_vec(:,iiuav) - eta0(:) - delta_eta_vec(:,iiuav));
for jjuav = 1:5
    ksi_est_err_tilt_4 = ksi_est_err_tilt_4 + ...
                                        wij(iiuav, jjuav) * ((ksi_d_est_vec(:,iiuav) - delta_ksi_vec(:,iiuav)) - (ksi_d_est_vec(:,jjuav) - delta_ksi_vec(:,jjuav)));
    eta_est_err_tilt_4 = eta_est_err_tilt_4 + ...
                                        wij(iiuav, jjuav) * ((eta_d_est_vec(:,iiuav) - delta_eta_vec(:,iiuav)) - (eta_d_est_vec(:,jjuav) - delta_eta_vec(:,jjuav)));
end

== matlab function sim_tcyb_2023_obs/cal lumped observation error agent 5 ==
  data: wij input; w0 input; ksi_d_est_vec input; ksi0 input; delta_ksi_vec input; eta_d_est_vec input; ksi_est_err_tilt_5 output; eta0 input; delta_eta_vec input; eta_est_err_tilt_5 output
function [ksi_est_err_tilt_5, eta_est_err_tilt_5]  = fcn(wij, w0, ksi_d_est_vec, ksi0, delta_ksi_vec, eta_d_est_vec, eta0, delta_eta_vec)
%%%% 计算跟随者期望速度分布式观测器误差
iiuav = 5;
ksi_est_err_tilt_5 = w0(iiuav, iiuav) * (ksi_d_est_vec(:,iiuav) - ksi0(:) - delta_ksi_vec(:,iiuav));
eta_est_err_tilt_5 = w0(iiuav, iiuav) * (eta_d_est_vec(:,iiuav) - eta0(:) - delta_eta_vec(:,iiuav));
for jjuav = 1:5
    ksi_est_err_tilt_5 = ksi_est_err_tilt_5 + ...
                                        wij(iiuav, jjuav) * ((ksi_d_est_vec(:,iiuav) - delta_ksi_vec(:,iiuav)) - (ksi_d_est_vec(:,jjuav) - delta_ksi_vec(:,jjuav)));
    eta_est_err_tilt_5 = eta_est_err_tilt_5 + ...
                                        wij(iiuav, jjuav) * ((eta_d_est_vec(:,iiuav) - delta_eta_vec(:,iiuav)) - (eta_d_est_vec(:,jjuav) - delta_eta_vec(:,jjuav)));
end

== matlab function sim_tcyb_2023_obs/cal position estimate error ==
  data: ksi_d_est_vec input; ksi_est_err output; ksi0 input; delta_ksi_vec input
function ksi_est_err  = fcn(ksi_d_est_vec, ksi0, delta_ksi_vec)
%%%% 计算跟随者期望位置分布式观测器误差
ksi_est_err = ksi_d_est_vec - repmat(ksi0, 1, 5) - delta_ksi_vec;

== matlab function sim_tcyb_2023_obs/cal velocity estimate error ==
  data: eta_d_est_vec input; eta_est_err output; eta0 input; delta_eta_vec input
function eta_est_err  = fcn(eta_d_est_vec, eta0, delta_eta_vec)
%%%% 计算跟随者期望速度分布式观测器误差
eta_est_err = eta_d_est_vec - repmat(eta0, 1, 5) - delta_eta_vec;

== matlab function sim_tcyb_2023_obs/combine follower desire velocity estimaters ==
  data: eta_d_est_1 input; eta_d_est_vec output; eta_d_est_2 input; eta_d_est_3 input; eta_d_est_4 input; eta_d_est_5 input
function eta_d_est_vec = fcn(eta_d_est_1, eta_d_est_2, eta_d_est_3, eta_d_est_4, eta_d_est_5)
%%%% 合并领导者位置观测器输出结果
eta_d_est_vec = [eta_d_est_1(:), eta_d_est_2(:), eta_d_est_3(:), eta_d_est_4(:), eta_d_est_5(:)];

== matlab function sim_tcyb_2023_obs/combine leader position estimaters ==
  data: ksi_d_est_1 input; ksi_d_est_vec output; ksi_d_est_2 input; ksi_d_est_3 input; ksi_d_est_4 input; ksi_d_est_5 input
function ksi_d_est_vec  = fcn(ksi_d_est_1, ksi_d_est_2, ksi_d_est_3, ksi_d_est_4, ksi_d_est_5)
%%%% 合并领导者位置观测器输出结果
ksi_d_est_vec = [ksi_d_est_1(:), ksi_d_est_2(:), ksi_d_est_3(:), ksi_d_est_4(:), ksi_d_est_5(:)];

== matlab function sim_tcyb_2023_obs/combine lumped follower observation error  ==
  data: ksi_est_err_tilt_1 input; ksi_est_err_tilt_2 input; ksi_est_err_tilt_3 input; ksi_est_err_tilt_4 input; ksi_est_err_tilt_5 input; ksi_est_err_tilt_vec output; eta_est_err_tilt_1 input; eta_est_err_tilt_vec output; eta_est_err_tilt_2 input; eta_est_err_tilt_3 input; eta_est_err_tilt_4 input; eta_est_err_tilt_5 input
function [ksi_est_err_tilt_vec, eta_est_err_tilt_vec]  = fcn(ksi_est_err_tilt_1, ksi_est_err_tilt_2, ksi_est_err_tilt_3, ksi_est_err_tilt_4, ksi_est_err_tilt_5, ...
                                                                                                        eta_est_err_tilt_1, eta_est_err_tilt_2, eta_est_err_tilt_3, eta_est_err_tilt_4, eta_est_err_tilt_5)
%%%% 合并领导者位置观测器输出结果
ksi_est_err_tilt_vec = [ksi_est_err_tilt_1, ksi_est_err_tilt_2, ksi_est_err_tilt_3, ksi_est_err_tilt_4, ksi_est_err_tilt_5];
eta_est_err_tilt_vec = [eta_est_err_tilt_1, eta_est_err_tilt_2, eta_est_err_tilt_3, eta_est_err_tilt_4, eta_est_err_tilt_5];

== matlab function sim_tcyb_2023_obs/divide eta_est_err ==
  data: eta_est_err input; eta_est_err_1 output; eta_est_err_2 output; eta_est_err_3 output; eta_est_err_4 output; eta_est_err_5 output
function [eta_est_err_1, eta_est_err_2, eta_est_err_3, eta_est_err_4, eta_est_err_5]  = fcn(eta_est_err)
%%%% 计算跟随者期望位置分布式观测器误差
eta_est_err_1 = eta_est_err(:,1);
eta_est_err_2 = eta_est_err(:,2);
eta_est_err_3 = eta_est_err(:,3);
eta_est_err_4 = eta_est_err(:,4);
eta_est_err_5 = eta_est_err(:,5);

== matlab function sim_tcyb_2023_obs/divide ksi_est_err ==
  data: ksi_est_err input; ksi_est_err_1 output; ksi_est_err_2 output; ksi_est_err_3 output; ksi_est_err_4 output; ksi_est_err_5 output
function [ksi_est_err_1, ksi_est_err_2, ksi_est_err_3, ksi_est_err_4, ksi_est_err_5]  = fcn(ksi_est_err)
%%%% 计算跟随者期望位置分布式观测器误差
ksi_est_err_1 = ksi_est_err(:,1);
ksi_est_err_2 = ksi_est_err(:,2);
ksi_est_err_3 = ksi_est_err(:,3);
ksi_est_err_4 = ksi_est_err(:,4);
ksi_est_err_5 = ksi_est_err(:,5);

== matlab function sim_tcyb_2023_obs/distributed follower desire velocity observer agent 1 ==
  data: c1 input; d_eta_d_est_1 output; eta_t input; u0 input; eta_est_err_tilt_vec input
function d_eta_d_est_1 = fcn(c1, eta_t, u0, eta_est_err_tilt_vec)
%%%% 跟随者期望速度分布式观测器
iiuav = 1;
d_eta_d_est_1 = u0(:) - 2 * ( eta_t + 2 ) * eta_est_err_tilt_vec(:,iiuav) ...
                                - c1 * ( eta_t + 2 ) * sign( eta_est_err_tilt_vec(:,iiuav) );

== matlab function sim_tcyb_2023_obs/generate function ksy_t d_ksy_t ==
  data: ts1 input; ksy_t output; ts2 input; tsim input; d_ksy_t output
function [ksy_t, d_ksy_t] = fcn(ts1, ts2, tsim)
%%%% 时域生成器
if tsim < ts1
    ksy_t = 10 * ( tsim ^ 6 ) / ( ts1 ^ 6 ) ...
                        - 24 * ( tsim ^ 5 ) / ( ts1 ^ 5 ) ...
                        + 15 * ( tsim ^ 4 ) / ( ts1 ^ 4 );
    d_ksy_t = 60 * ( tsim ^ 5 ) / ( ts1 ^ 6 ) ...
                        - 120 * ( tsim ^ 4 ) / ( ts1 ^ 5 ) ...
                        + 60 * ( tsim ^ 3 ) / ( ts1 ^ 4 );
elseif tsim < ts2
    ksy_t = 10 * ( tsim ^ 6 ) / ( ts2 ^ 6 ) ...
                        - 24 * ( tsim ^ 5 ) / ( ts2 ^ 5 ) ...
                        + 15 * ( tsim ^ 4 ) / ( ts2 ^ 4 );
    d_ksy_t = 60 * ( tsim ^ 5 ) / ( ts2 ^ 6 ) ...
                        - 120 * ( tsim ^ 4 ) / ( ts2 ^ 5 ) ...
                        + 60 * ( tsim ^ 3 ) / ( ts2 ^ 4 );
else
    ksy_t = 1;
    d_ksy_t = 0;
end

== matlab function sim_tcyb_2023_obs/generate function h_t ==
  data: k0 input; ts1 input; h_t output; ts2 input; delta1 input; delta2 input; tsim input; ksy_t input; d_ksy_t input
function h_t = fcn(k0, ts1, ts2, delta1, delta2, tsim, ksy_t, d_ksy_t)
%%%% 构造函数
if tsim < ts1
    h_t = ( k0 * d_ksy_t ) / ( 1 - ksy_t + delta1 );
elseif tsim < ts2
    h_t = ( k0 * d_ksy_t ) / ( 1 - ksy_t + delta2 );
else
    h_t = 0;
end

== matlab function sim_tcyb_2023_obs/generate function eta_t ==
  data: lambda_max_P input; eta_t output; lambda_min_Q input; h_t input
function eta_t = fcn(lambda_max_P, lambda_min_Q, h_t)
%%%% 观测器系数
eta_t = ( lambda_max_P / ( 2 * lambda_min_Q ) ) * h_t;

== matlab function sim_tcyb_2023_obs/leader control input ==
  data: t input; u0 output; T1 input; T2 input; R0 input; R1 input; Rx2 input; Ry2 input; Rz2 input
function u0  = fcn(t, T1, T2, R0, R1, Rx2, Ry2, Rz2)
%%%% 给出领导者参考加速度控制输入
u0 = zeros(3, 1);

if t <= ( T1 + 1e-05 )
    u0(1, 1) = - ( 4 * pi * sin( ( 2 * pi * ( t - 0 ) ) / ( 0 - T1 ) ) * ( R0 - R1 ) ) / ( ( 0 - T1 ) ^ 2 ) ...
                        - ( 4 * ( pi ^ 2 ) * cos( ( 2 * pi * ( t - 0 ) ) / ( 0 - T1 ) ) ...
                        * ( R0 + ( ( R0 - R1 ) * ( t - 0 ) ) / ( 0 - T1 ) ) ) / ( ( 0 - T1 ) ^ 2 );
    u0(2, 1) = ( 4 * pi * cos( ( 2 * pi * ( t - 0 ) ) / ( 0 - T1 ) ) * ( R0 - R1 ) ) / ( ( 0 - T1 ) ^ 2 ) ...
                        - ( 4 * ( pi ^ 2 ) * sin( ( 2 * pi * ( t - 0 ) ) / ( 0 - T1 ) ) ...
                        * ( R0 + ( ( R0 - R1 ) * ( t - 0 ) ) / ( 0 - T1 ) ) ) / ( ( 0 - T1 ) ^ 2 );
    u0(3, 1) = 0;
else
    u0(1, 1) = ( 4 * Rx2 * ( pi ^ 2 ) * cos( ( 2 * pi * ( t - T1 ) ) / ( T1 - T2 ) ) ) / ( ( T1 - T2 ) ^ 2 );
    u0(2, 1) = - ( 16 * Ry2 * ( pi ^ 2 ) * sin( ( 4 * pi * ( t - T1 ) ) / ( T1 - T2 ) ) ) / ( ( T1 - T2 ) ^ 2 );
    u0(3, 1) = ( 16 * Rz2 * ( pi ^ 2 ) * sin( ( 4 * pi * ( t - T1 ) ) / ( T1 - T2 ) ) ) / ( ( T1 - T2 ) ^ 2 );
end
